simulink model "cvoo_g19_falta_ficar_bonito_2020a"  (R2021a)
settings: Solver=VariableStepAuto  StartTime=0.0  StopTime=100  RelTol=1e-3
values from neighbouring files (symbols this model uses):
  b_h_pt = [ ... (first row only)    [Ponto3.m]    (also in main.m; main_novo.m)
  c_h_pt = eye(size(a_h_pt))    [Ponto3.m]    (also in main.m; main_novo.m)
  conv_max = 5    [main.m]    (also in main_novo.m)
  conv_min = 0    [main.m]    (also in main_novo.m)
  conv_rms = 1.5*conv_res    (= 0.000915639116103)    [main.m]    (also in main_novo.m = 0.0018310546875)
  d_h_pt = zeros(size(b_h_pt))    [Ponto3.m]    (also in main.m; main_novo.m)
  deg = pi/180    (= 0.0174532925199)    [Ponto3.m]    (also in def_model.m; def_model_inicial.m; main.m; main_controlo_altitude.m)
  f_amost = 100    [main.m]    (also in main_novo.m)
  fat_conv_ra = 1/3    (= 0.333333333333)    [main_novo.m]
  G_ra = 10e-3/ft    (= 0.0328083989501)    [main_novo.m]
  G_sensq = (V_max_sensq-V_min_sensq)/(q_max_sensq-q_min_sensq)    (= 0.006)    [main.m]    (also in main_novo.m)
  Gp_din = (v_pdin_max-v_pdin_min)/(pdin_max-pdin_min)    (= 0.00125)    [main.m]    (also in main_novo.m)
  h_ra_max = 1500*ft    (= 457.2)    [main_novo.m]
  h_ra_min = 0    [main_novo.m]
  h_seguimento = 100    [main_novo.m]
  h_solo_0 = 5* cond_ini.u0+100    [main_novo.m]
  K_lqr = lqr(a_h_pt_int, b_h_pt_int, Q, R)    [Ponto3.m]    (also in main.m; main_controlo_altitude.m = lqr(a_h_int, b_h_sf_int, Q, R); main_novo.m)
  offset_pdin = 2.5    [main.m]    (also in main_novo.m)
  Offset_ra = 0    [main_novo.m]
  Offset_sensq = 2.5    [main.m]    (also in main_novo.m)
  p_din_tau = 0.01    [main.m]    (also in main_novo.m)
  pdin_max = 2e3    (= 2000)    [main.m]    (also in main_novo.m)
  pdin_min = -2e3    (= -2000)    [main.m]    (also in main_novo.m)
  q_max_sensq = 300    [main.m]    (also in main_novo.m)
  q_min_sensq = -300    [main.m]    (also in main_novo.m)
  ra_rms = 0.015    [main_novo.m]
  rad = 180/pi    (= 57.2957795131)    [Ponto3.m]    (also in main.m; main_controlo_altitude.m; main_novo.m)
  rho0 = 1.225    [main.m]    (also in main_novo.m)
  rms_sensq = 4.4    [main.m]    (also in main_novo.m)
  tau = 0.1    [main.m]    (also in main_novo.m)
  u_ref = 1.5    [Ponto3.m]    (also in main.m = 2; main_controlo_altitude.m = -5; main_novo.m = 0)
  vel_max_at = 60    [main.m]    (also in main_novo.m)
  vel_vento = 10    [main_novo.m]
  x0 = [0 0 0 0]    [Ponto3.m]    (also in main.m; main_controlo_altitude.m; main_novo.m)
  x0_e = [0 0 0 0 cond_ini.h0+h_solo_0]    [main_novo.m]
undefined symbols (not defined in the file or in its folder): a_h_pt, ae, be, ce, cond_ini, de, max_deflec
libraries: simulink x5
settings Model: Creator=josem  LastModifiedBy=thomasmchilds
settings SolverCC: AlgebraicLoopSolver=TrustRegion
settings DebuggingCC: SFMachineParentedDataDiag=warning

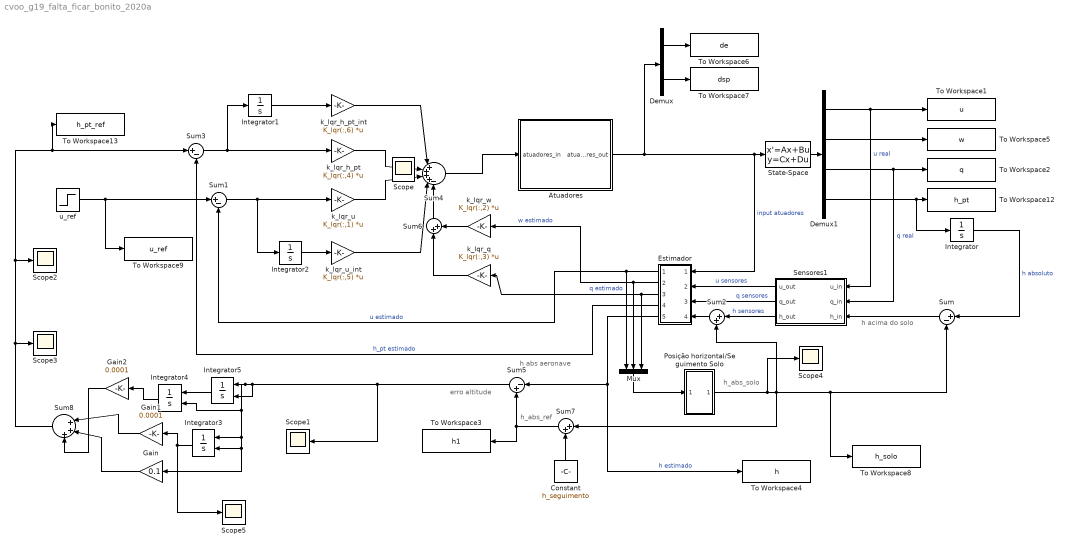
== system cvoo_g19_falta_ficar_bonito_2020a ==
  note: erro altitude
  note: h_abs_solo
  note: h_abs_ref
  note: h abs aeronave
  note: h acima do solo
  Atuadores : Subsystem
  Constant : Constant  Value=h_seguimento
  Demux : Demux  Outputs=2
  Demux1 : Demux
  Estimador : Subsystem
  Gain : Gain  Gain=0.1
  Gain1 : Gain  Gain=0.0001
  Gain2 : Gain  Gain=0.0001
  Integrator : Integrator  InitialCondition=cond_ini.h0+h_solo_0
  Integrator1 : Integrator
  Integrator2 : Integrator
  Integrator3 : Integrator  ExternalReset=either
  Integrator4 : Integrator  ExternalReset=either
  Integrator5 : Integrator  ExternalReset=either
  Mux : Mux  Inputs=3
  Posição horizontal/Seguimento Solo : Subsystem
  Scope{,1..5} (6 alike) : Scope
  Sensores1 : Subsystem
  State-Space : StateSpace  A=a_h_pt  B=b_h_pt  C=c_h_pt  D=d_h_pt  InitialCondition=x0
  Sum : Sum  Inputs=|+-
  Sum1 : Sum  Inputs=|+-
  Sum2 : Sum  Inputs=|++
  Sum3 : Sum  Inputs=|+-
  Sum4 : Sum  Inputs=|++++-
  Sum5 : Sum  Inputs=|-+
  Sum6 : Sum  Inputs=|++
  Sum7 : Sum  Inputs=|++
  Sum8 : Sum  Inputs=|+++
  To Workspace1 : ToWorkspace  VariableName=u  SampleTime=-1
  To Workspace12 : ToWorkspace  VariableName=h_pt  SampleTime=-1
  To Workspace13 : ToWorkspace  VariableName=h_pt_ref  SampleTime=-1
  To Workspace2 : ToWorkspace  VariableName=q  SampleTime=-1
  To Workspace3 : ToWorkspace  VariableName=h1  SampleTime=-1
  To Workspace4 : ToWorkspace  VariableName=h  SampleTime=-1
  To Workspace5 : ToWorkspace  VariableName=w  SampleTime=-1
  To Workspace6 : ToWorkspace  VariableName=de  SaveFormat=Structure With Time  SampleTime=-1
  To Workspace7 : ToWorkspace  VariableName=dsp  SaveFormat=Structure With Time  SampleTime=-1
  To Workspace8 : ToWorkspace  VariableName=h_solo  SampleTime=-1
  To Workspace9 : ToWorkspace  VariableName=u_ref  SampleTime=-1
  k_lqr_h_pt : Gain  Gain=K_lqr(:,4)  Multiplication=Matrix(K*u)
  k_lqr_h_pt_int : Gain  Gain=K_lqr(:,6)  Multiplication=Matrix(K*u)
  k_lqr_q : Gain  Gain=K_lqr(:,3)  Multiplication=Matrix(K*u)
  k_lqr_u : Gain  Gain=K_lqr(:,1)  Multiplication=Matrix(K*u)
  k_lqr_u_int : Gain  Gain=K_lqr(:,5)  Multiplication=Matrix(K*u)
  k_lqr_w : Gain  Gain=K_lqr(:,2)  Multiplication=Matrix(K*u)
  u_ref : Step  After=u_ref  SampleTime=0
  wires:
  State-Space/1 -> Demux1/1
  Demux1/2 -> To Workspace5/1
  k_lqr_h_pt/1 -> Sum4/2
  k_lqr_w/1 -> Sum6/2
  k_lqr_q/1 -> Sum6/1
  Sum6/1 -> Sum4/5
  Demux/1 -> To Workspace6/1
  Demux/2 -> To Workspace7/1
  Demux1/4 -> Integrator/1, To Workspace12/1
  Demux1/1 -> Sensores1/1(u_in), To Workspace1/1  "u real"
  k_lqr_u/1 -> Sum4/3
  Sum3/1 -> Integrator1/1, k_lqr_h_pt/1
  Integrator1/1 -> k_lqr_h_pt_int/1
  k_lqr_h_pt_int/1 -> Sum4/1
  k_lqr_u_int/1 -> Sum4/4
  Sum1/1 -> Integrator2/1, k_lqr_u/1
  Integrator2/1 -> k_lqr_u_int/1
  Atuadores/1(atuadores_out) -> State-Space/1, Estimador/1(In1), Demux/1  "input atuadores"
  Demux1/3 -> Sensores1/2(q_in), To Workspace2/1  "q real"
  Integrator/1 -> Sum/1  "h absoluto"
  Estimador/4(Out1) -> Sum3/2  "h_pt estimado"
  Estimador/3(Out3) -> Mux/3, k_lqr_q/1  "q estimado"
  Sensores1/1(u_out) -> Estimador/2(In2)  "u sensores"
  Sensores1/2(q_out) -> Estimador/3(In3)  "q sensores"
  Sum/1 -> Sensores1/3(h_in)
  Posição horizontal/Seguimento Solo/1(Out1) -> Scope4/1, Sum2/2, Sum/2, To Workspace8/1, Sum7/1
  Estimador/2(Out2) -> Mux/2, k_lqr_w/1  "w estimado"
  Estimador/1(Out4) -> Mux/1, Sum1/2  "u estimado"
  Mux/1 -> Posição horizontal/Seguimento Solo/1(In1)
  Sum2/1 -> Estimador/4(In4)
  Sensores1/3(h_out) -> Sum2/1  "h sensores"
  Estimador/5(Out5) -> To Workspace4/1, Sum5/1  "h estimado"
  Sum7/1 -> To Workspace3/1, Sum5/2
  Constant/1 -> Sum7/2
  Integrator3/1 -> Gain1/1, Scope5/1
  Gain/1 -> Sum8/2
  u_ref/1 -> To Workspace9/1, Sum1/1
  Sum8/1 -> Scope3/1, Scope2/1, To Workspace13/1, Sum3/1
  Gain1/1 -> Sum8/1
  Sum5/1 -> Scope1/1, Integrator5/2, Integrator5/1, Integrator4/2, Integrator3/2, Gain/1, Integrator3/1
  Gain2/1 -> Sum8/3
  Integrator5/1 -> Integrator4/1
  Integrator4/1 -> Gain2/1
  Sum4/1 -> Atuadores/1(atuadores_in)

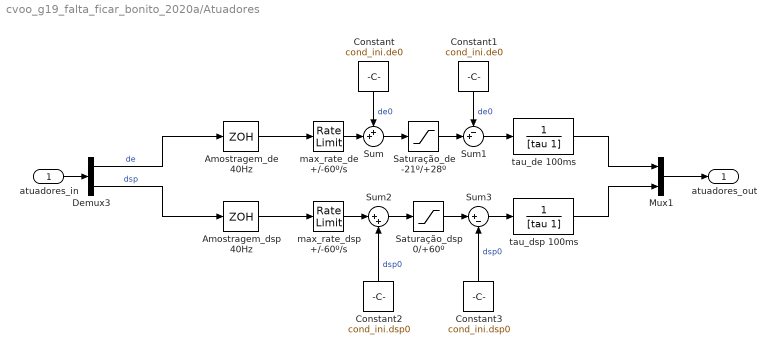
== system cvoo_g19_falta_ficar_bonito_2020a/Atuadores ==
  atuadores_in : Inport
  " max_rate_de +/-60º/s" : RateLimiter  RisingSlewLimit=vel_max_at*deg  FallingSlewLimit=-vel_max_at*deg  SampleTimeMode=inherited
  " max_rate_dsp +/-60º/s" : RateLimiter  RisingSlewLimit=vel_max_at*deg  FallingSlewLimit=-vel_max_at*deg  SampleTimeMode=inherited
  Amostragem_de 40Hz : ZeroOrderHold  SampleTime=1/f_amost
  Amostragem_dsp 40Hz : ZeroOrderHold  SampleTime=1/f_amost
  Constant : Constant  Value=cond_ini.de0
  Constant1 : Constant  Value=cond_ini.de0
  Constant2 : Constant  Value=cond_ini.dsp0
  Constant3 : Constant  Value=cond_ini.dsp0
  Demux3 : Demux  Outputs=2
  Mux1 : Mux  Inputs=2
  Saturação_de -21º/+28º : Saturate  UpperLimit=max_deflec.demax  LowerLimit=max_deflec.demin
  Saturação_dsp 0/+60º : Saturate  UpperLimit=max_deflec.spmax  LowerLimit=0
  Sum : Sum  Inputs=++|
  Sum1 : Sum  Inputs=-+|
  Sum2 : Sum  Inputs=|++
  Sum3 : Sum  Inputs=|+-
  tau_de 100ms : TransferFcn  Denominator=[tau 1]
  tau_dsp 100ms : TransferFcn  Denominator=[tau 1]
  atuadores_out : Outport
  wires:
  Mux1/1 -> atuadores_out/1
  atuadores_in/1 -> Demux3/1
  Demux3/1 -> Amostragem_de 40Hz/1  "de"
  Demux3/2 -> Amostragem_dsp 40Hz/1  "dsp"
  tau_dsp 100ms/1 -> Mux1/2
  tau_de 100ms/1 -> Mux1/1
  Amostragem_dsp 40Hz/1 -> " max_rate_dsp +/-60º/s"/1
  Amostragem_de 40Hz/1 -> " max_rate_de +/-60º/s"/1
  " max_rate_de +/-60º/s"/1 -> Sum/2
  Sum/1 -> Saturação_de -21º/+28º/1
  Constant/1 -> Sum/1  "de0"
  Saturação_de -21º/+28º/1 -> Sum1/2
  Sum1/1 -> tau_de 100ms/1
  Constant1/1 -> Sum1/1  "de0"
  " max_rate_dsp +/-60º/s"/1 -> Sum2/1
  Sum2/1 -> Saturação_dsp 0/+60º/1
  Constant2/1 -> Sum2/2  "dsp0"
  Constant3/1 -> Sum3/2  "dsp0"
  Saturação_dsp 0/+60º/1 -> Sum3/1
  Sum3/1 -> tau_dsp 100ms/1

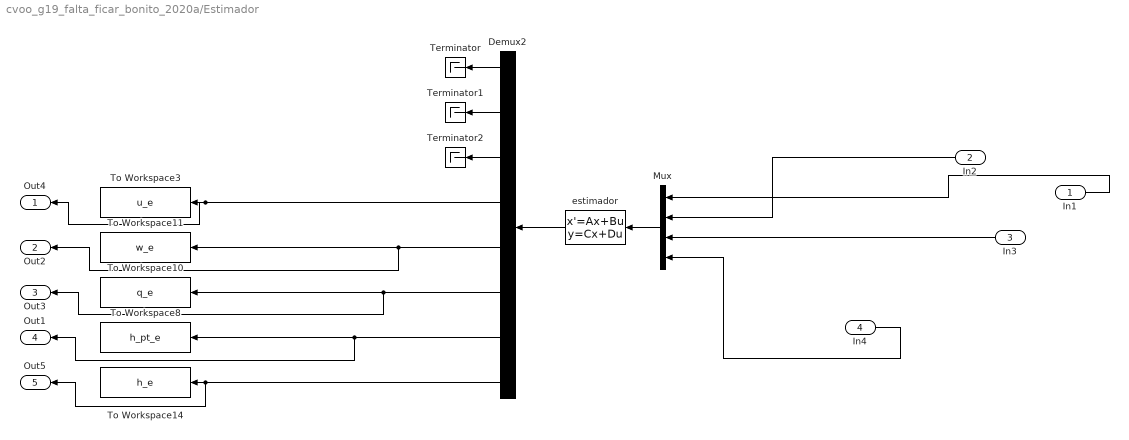
== system cvoo_g19_falta_ficar_bonito_2020a/Estimador ==
  In1 : Inport
  In2 : Inport  Port=2
  In3 : Inport  Port=3
  In4 : Inport  Port=4
  Demux2 : Demux  Outputs=8
  Mux : Mux
  Terminator : Terminator
  Terminator1 : Terminator
  Terminator2 : Terminator
  To Workspace10 : ToWorkspace  VariableName=q_e  SampleTime=-1
  To Workspace11 : ToWorkspace  VariableName=w_e  SampleTime=-1
  To Workspace14 : ToWorkspace  VariableName=h_e  SampleTime=-1
  To Workspace3 : ToWorkspace  VariableName=u_e  SampleTime=-1
  To Workspace8 : ToWorkspace  VariableName=h_pt_e  SampleTime=-1
  estimador : StateSpace  A=ae  B=be  C=ce  D=de  InitialCondition=x0_e
  Out4 : Outport
  Out2 : Outport  Port=2
  Out3 : Outport  Port=3
  Out1 : Outport  Port=4
  Out5 : Outport  Port=5
  wires:
  Demux2/2 -> Terminator1/1
  estimador/1 -> Demux2/1
  Demux2/5 -> Out2/1, To Workspace11/1
  Demux2/7 -> Out1/1, To Workspace8/1
  Demux2/8 -> Out5/1, To Workspace14/1
  Demux2/1 -> Terminator/1
  Demux2/4 -> Out4/1, To Workspace3/1
  Demux2/3 -> Terminator2/1
  Mux/1 -> estimador/1
  Demux2/6 -> Out3/1, To Workspace10/1
  In1/1 -> Mux/1
  In3/1 -> Mux/3
  In2/1 -> Mux/2
  In4/1 -> Mux/4

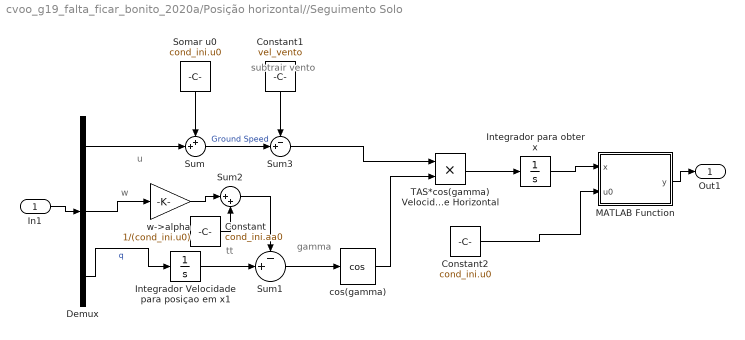
== system cvoo_g19_falta_ficar_bonito_2020a/Posição horizontal//Seguimento Solo ==
  note: subtrair vento
  note: w
  note: tt
  note: u
  note: gamma
  In1 : Inport
  Constant : Constant  Value=cond_ini.aa0
  Constant1 : Constant  Value=vel_vento
  Constant2 : Constant  Value=cond_ini.u0
  Demux : Demux  Outputs=3
  Integrador para obter x : Integrator
  Integrador Velocidade para posiçao em x1 : Integrator  InitialCondition=cond_ini.tt0
  MATLAB Function : MATLAB Function  TreatAsAtomicUnit=on
  Somar u0 : Constant  Value=cond_ini.u0
  Sum : Sum  Inputs=++|
  Sum1 : Sum  Inputs=-+|
  Sum2 : Sum  Inputs=|++
  Sum3 : Sum  Inputs=-+|
  TAS*cos(gamma) Velocidade Horizontal : Product
  cos(gamma) : Trigonometry  Operator=cos
  w->alpha : Gain  Gain=1/(cond_ini.u0)
  Out1 : Outport  VectorParamsAs1DForOutWhenUnconnected=off
  wires:
  In1/1 -> Demux/1
  Demux/1 -> Sum/2
  Demux/2 -> w->alpha/1
  Demux/3 -> Integrador Velocidade para posiçao em x1/1  "q"
  Sum1/1 -> cos(gamma)/1
  cos(gamma)/1 -> TAS*cos(gamma) Velocidade Horizontal/2
  MATLAB Function/1(y) -> Out1/1
  Sum2/1 -> Sum1/1
  Constant/1 -> Sum2/2
  w->alpha/1 -> Sum2/1
  Integrador Velocidade para posiçao em x1/1 -> Sum1/2
  Somar u0/1 -> Sum/1
  Sum/1 -> Sum3/2  "Ground Speed"
  Constant1/1 -> Sum3/1
  Sum3/1 -> TAS*cos(gamma) Velocidade Horizontal/1
  Constant2/1 -> MATLAB Function/2(u0)
  Integrador para obter x/1 -> MATLAB Function/1(x)
  TAS*cos(gamma) Velocidade Horizontal/1 -> Integrador para obter x/1

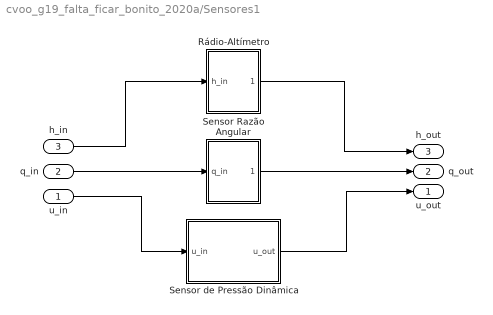
== system cvoo_g19_falta_ficar_bonito_2020a/Sensores1 ==
  u_in : Inport
  q_in : Inport  Port=2
  h_in : Inport  Port=3
  Rádio-Altímetro : Subsystem
  Sensor Razão Angular : Subsystem
  Sensor de Pressão Dinâmica : Subsystem
  u_out : Outport
  q_out : Outport  Port=2
  h_out : Outport  Port=3
  wires:
  Sensor Razão Angular/1(q_out) -> q_out/1
  u_in/1 -> Sensor de Pressão Dinâmica/1(u_in)
  Sensor de Pressão Dinâmica/1(u_out) -> u_out/1
  q_in/1 -> Sensor Razão Angular/1(q_in)
  h_in/1 -> Rádio-Altímetro/1(h_in)
  Rádio-Altímetro/1(h_out) -> h_out/1

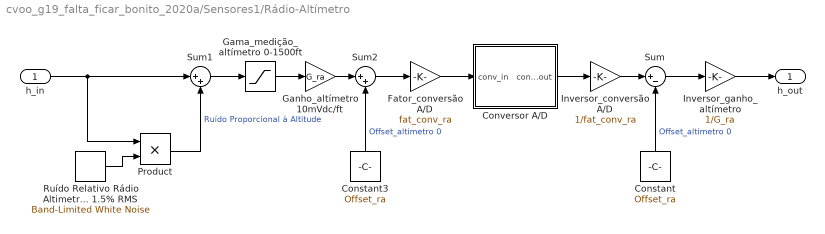
== system cvoo_g19_falta_ficar_bonito_2020a/Sensores1/Rádio-Altímetro ==
  h_in : Inport
  Constant : Constant  Value=Offset_ra
  Constant3 : Constant  Value=Offset_ra
  Conversor A/D : Subsystem
  Fator_conversão A/D : Gain  Gain=fat_conv_ra
  Gama_medição_altímetro 0-1500ft : Saturate  UpperLimit=h_ra_max  LowerLimit=h_ra_min
  Ganho_altímetro 10mVdc/ft : Gain  Gain=G_ra
  Inversor_conversão A/D : Gain  Gain=1/fat_conv_ra
  Inversor_ganho_altímetro : Gain  Gain=1/G_ra
  Product : Product
  Ruído Relativo Rádio Altimetro 1.5% RMS : simulink/Sources/Band-Limited White Noise  Cov=[ra_rms^2/f_amost]  Ts=1/f_amost  seed=[23341]
  Sum : Sum  Inputs=|+-
  Sum1 : Sum  Inputs=|++
  Sum2 : Sum  Inputs=|++
  h_out : Outport
  wires:
  Sum/1 -> Inversor_ganho_altímetro/1
  Constant/1 -> Sum/2  "Offset_altimetro 0"
  Sum2/1 -> Fator_conversão A/D/1
  Fator_conversão A/D/1 -> Conversor A/D/1(conv_in)
  Inversor_conversão A/D/1 -> Sum/1
  Conversor A/D/1(conv_out) -> Inversor_conversão A/D/1
  Inversor_ganho_altímetro/1 -> h_out/1
  h_in/1 -> Product/1, Sum1/1
  Sum1/1 -> Gama_medição_altímetro 0-1500ft/1
  Ganho_altímetro 10mVdc/ft/1 -> Sum2/1
  Gama_medição_altímetro 0-1500ft/1 -> Ganho_altímetro 10mVdc/ft/1
  Constant3/1 -> Sum2/2  "Offset_altimetro 0"
  Ruído Relativo Rádio Altimetro 1.5% RMS/1 -> Product/2
  Product/1 -> Sum1/2  "Ruído Proporcional à Altitude"

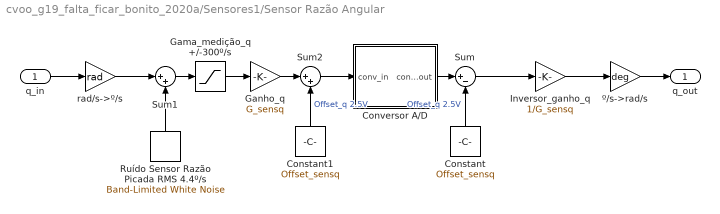
== system cvoo_g19_falta_ficar_bonito_2020a/Sensores1/Sensor Razão Angular ==
  q_in : Inport
  Constant : Constant  Value=Offset_sensq
  Constant1 : Constant  Value=Offset_sensq
  Conversor A/D : Subsystem
  Gama_medição_q +/-300º/s : Saturate  UpperLimit=q_max_sensq  LowerLimit=q_min_sensq
  Ganho_q : Gain  Gain=G_sensq
  Inversor_ganho_q : Gain  Gain=1/G_sensq
  Ruído Sensor Razão Picada RMS 4.4º/s : simulink/Sources/Band-Limited White Noise  Cov=[rms_sensq^2/f_amost]  Ts=1/f_amost  seed=[23341]
  Sum : Sum  Inputs=|+-
  Sum1 : Sum  Inputs=|++
  Sum2 : Sum  Inputs=|++
  rad/s->º/s : Gain  Gain=rad
  º/s->rad/s : Gain  Gain=deg
  q_out : Outport
  wires:
  Conversor A/D/1(conv_out) -> Sum/1
  Sum/1 -> Inversor_ganho_q/1
  Constant/1 -> Sum/2  "Offset_q 2.5V"
  Inversor_ganho_q/1 -> º/s->rad/s/1
  º/s->rad/s/1 -> q_out/1
  Sum1/1 -> Gama_medição_q +/-300º/s/1
  Gama_medição_q +/-300º/s/1 -> Ganho_q/1
  rad/s->º/s/1 -> Sum1/1
  Constant1/1 -> Sum2/2  "Offset_q 2.5V"
  Ganho_q/1 -> Sum2/1
  Ruído Sensor Razão Picada RMS 4.4º/s/1 -> Sum1/2
  q_in/1 -> rad/s->º/s/1
  Sum2/1 -> Conversor A/D/1(conv_in)

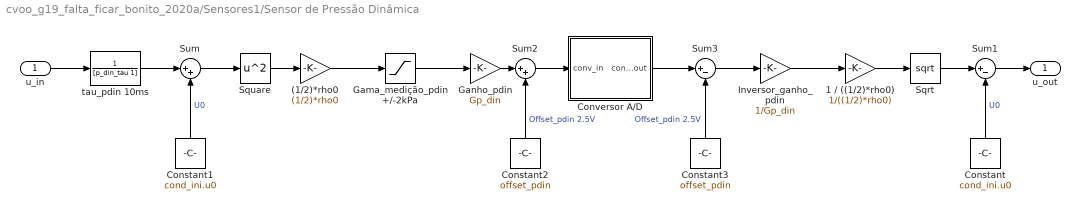
== system cvoo_g19_falta_ficar_bonito_2020a/Sensores1/Sensor de Pressão Dinâmica ==
  u_in : Inport
  (1/2)*rho0 : Gain  Gain=(1/2)*rho0
  1 / ((1/2)*rho0) : Gain  Gain=1/((1/2)*rho0)
  Constant : Constant  Value=cond_ini.u0
  Constant1 : Constant  Value=cond_ini.u0
  Constant2 : Constant  Value=offset_pdin
  Constant3 : Constant  Value=offset_pdin
  Conversor A/D : Subsystem
  Gama_medição_pdin +/-2kPa : Saturate  UpperLimit=pdin_max  LowerLimit=pdin_min
  Ganho_pdin : Gain  Gain=Gp_din
  Inversor_ganho_pdin : Gain  Gain=1/Gp_din
  Sqrt : Sqrt  SaturateOnIntegerOverflow=on
  Square : Math  Operator=square  SignedPower=on  SaturateOnIntegerOverflow=on
  Sum : Sum  Inputs=|++
  Sum1 : Sum  Inputs=|+-
  Sum2 : Sum  Inputs=|++
  Sum3 : Sum  Inputs=|+-
  tau_pdin 10ms : TransferFcn  Denominator=[p_din_tau 1]
  u_out : Outport
  wires:
  u_in/1 -> tau_pdin 10ms/1
  Sum/1 -> Square/1
  Ganho_pdin/1 -> Sum2/1
  Constant2/1 -> Sum2/2  "Offset_pdin 2.5V"
  tau_pdin 10ms/1 -> Sum/1
  (1/2)*rho0/1 -> Gama_medição_pdin +/-2kPa/1
  Constant1/1 -> Sum/2  "U0"
  Gama_medição_pdin +/-2kPa/1 -> Ganho_pdin/1
  Square/1 -> (1/2)*rho0/1
  Sum2/1 -> Conversor A/D/1(conv_in)
  Constant/1 -> Sum1/2  "U0"
  Sqrt/1 -> Sum1/1
  1 / ((1/2)*rho0)/1 -> Sqrt/1
  Inversor_ganho_pdin/1 -> 1 / ((1/2)*rho0)/1
  Sum3/1 -> Inversor_ganho_pdin/1
  Conversor A/D/1(conv_out) -> Sum3/1
  Sum1/1 -> u_out/1
  Constant3/1 -> Sum3/2  "Offset_pdin 2.5V"

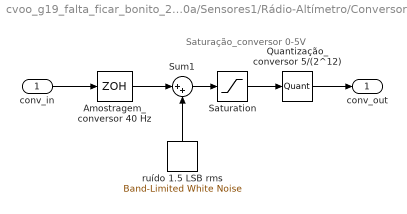
== system cvoo_g19_falta_ficar_bonito_2020a/Sensores1/Rádio-Altímetro/Conversor A//D ==
  note: Saturação_conversor
      |               0-5V
  conv_in : Inport
  Amostragem_conversor 40 Hz : ZeroOrderHold  SampleTime=1/f_amost
  Quantização_conversor 5/(2^12) : Quantizer  QuantizationInterval=fat_quant
  Saturation : Saturate  UpperLimit=conv_max  LowerLimit=conv_min
  Sum1 : Sum  Inputs=|++
  ruído 1.5 LSB rms : simulink/Sources/Band-Limited White Noise  Cov=[conv_rms^2/f_amost]  Ts=1/f_amost  seed=[23341]
  conv_out : Outport
  wires:
  conv_in/1 -> Amostragem_conversor 40 Hz/1
  Amostragem_conversor 40 Hz/1 -> Sum1/1
  ruído 1.5 LSB rms/1 -> Sum1/2
  Saturation/1 -> Quantização_conversor 5/(2^12)/1
  Sum1/1 -> Saturation/1
  Quantização_conversor 5/(2^12)/1 -> conv_out/1

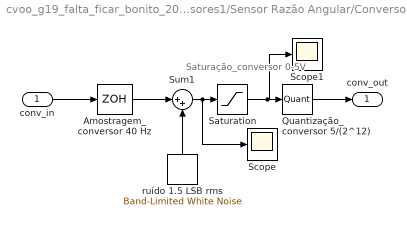
== system cvoo_g19_falta_ficar_bonito_2020a/Sensores1/Sensor Razão Angular/Conversor A//D ==
  note: Saturação_conversor
      |               0-5V
  conv_in : Inport
  Amostragem_conversor 40 Hz : ZeroOrderHold  SampleTime=1/f_amost
  Quantização_conversor 5/(2^12) : Quantizer  QuantizationInterval=fat_quant
  Saturation : Saturate  UpperLimit=conv_max  LowerLimit=conv_min
  Scope : Scope
  Scope1 : Scope
  Sum1 : Sum  Inputs=|++
  ruído 1.5 LSB rms : simulink/Sources/Band-Limited White Noise  Cov=[conv_rms^2/f_amost]  Ts=1/f_amost  seed=[23341]
  conv_out : Outport
  wires:
  conv_in/1 -> Amostragem_conversor 40 Hz/1
  Amostragem_conversor 40 Hz/1 -> Sum1/1
  ruído 1.5 LSB rms/1 -> Sum1/2
  Saturation/1 -> Scope1/1, Quantização_conversor 5/(2^12)/1
  Sum1/1 -> Scope/1, Saturation/1
  Quantização_conversor 5/(2^12)/1 -> conv_out/1

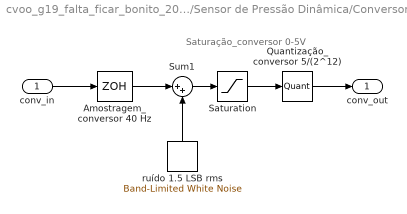
== system cvoo_g19_falta_ficar_bonito_2020a/Sensores1/Sensor de Pressão Dinâmica/Conversor A//D ==
  note: Saturação_conversor
      |               0-5V
  conv_in : Inport
  Amostragem_conversor 40 Hz : ZeroOrderHold  SampleTime=1/f_amost
  Quantização_conversor 5/(2^12) : Quantizer  QuantizationInterval=fat_quant
  Saturation : Saturate  UpperLimit=conv_max  LowerLimit=conv_min
  Sum1 : Sum  Inputs=|++
  ruído 1.5 LSB rms : simulink/Sources/Band-Limited White Noise  Cov=[conv_rms^2/f_amost]  Ts=1/f_amost  seed=[23341]
  conv_out : Outport
  wires:
  conv_in/1 -> Amostragem_conversor 40 Hz/1
  Amostragem_conversor 40 Hz/1 -> Sum1/1
  ruído 1.5 LSB rms/1 -> Sum1/2
  Saturation/1 -> Quantização_conversor 5/(2^12)/1
  Sum1/1 -> Saturation/1
  Quantização_conversor 5/(2^12)/1 -> conv_out/1

== matlab function cvoo_g19_falta_ficar_bonito_2020a/Posição horizontal//Seguimento Solo/MATLAB Function ==
  data: x input; y output; u0 input
function y = fcn(x, u0)

% if (u<20*u0)
%    y=(-5/20)*u+5*u0;
% elseif (20*u0<=u) && (u<40*u0)
%    y=0;
% elseif (40*u0<=u) && (u<60*u0)
%    %y=2.5*u0*sin((3.14159265359/(20*u0))*u) +2.5*u0;
%    y=5*u0*sin(((u/(20*u0))-2)*pi/2);
% 
% else
%     
%    y=5*u0;

if (x<40*u0)
   y=(-5/40)*x+5*u0+100;
   
elseif (40*u0<=x) && (x<60*u0)
   y=100;
   
elseif (60*u0<=x) && (x<100*u0)
   %y=2.5*u0*sin((3.14159265359/(20*u0))*u) +2.5*u0;
   %y=5*u0*sin(((u/(20*u0))-2)*pi/2);
   amplitude = 50; %(m)
   periodo = 40*2; %meio periodo sao 40s
   offset = +50;
   y=offset+amplitude*sin(2*pi/(periodo*u0)*(x-60*u0)+pi/2);

else
    
   y=0;
end
